simulink model "SZAU"  (R2017b)
settings: Solver=VariableStepAuto  StartTime=0.0  StopTime=1000  RelTol=1e-3
values from neighbouring files (symbols this model uses):
  A1 = 505    [SZAU_lin.mat]
  a1 = 22    [SZAU_lin.mat]
  a2 = 16    [SZAU_lin.mat]
  C2 = 0.65    [SZAU_lin.mat]
  Fd = 13    [SZAU_lin.mat]
  h10 = 17.87    [SZAU_lin.mat]
  h20 = 33.7852    [SZAU_lin.mat]
  tau = 80    [SZAU_lin.mat]
libraries: mpclib x1
settings Model: Creator=Jarzyn  LastModifiedBy=Jarzyn

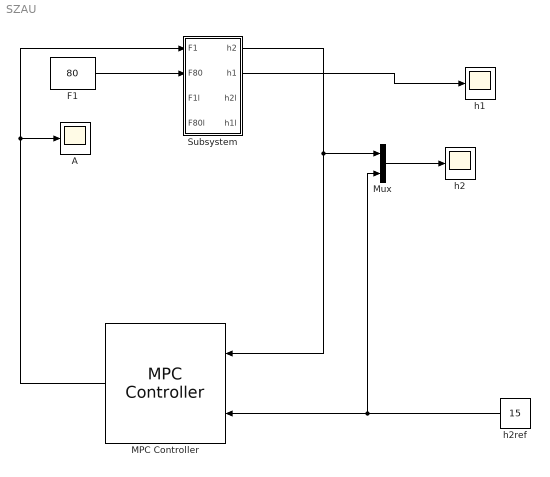
== system SZAU ==
  A : Scope
  F1 : Constant  Value=80  SampleTime=0
  MPC Controller : mpclib/MPC Controller  SCDEnableBlockLinearizationSpecification=on  mpcobj=mpc1  is_multiple=0  enable_value=0  return_u0=off  ref_from_ws=off  ref_signal_name=[]  ref_preview=off  md_from_ws=off  md_signal_name=[]  md_preview=off  from_project=off  project_file=MPCtask.mat  md_inport=off  mv_inport=off  cost_outport=off  return_sequence=off  return_qpstatus=off  return_state=off  state_inport=off  lims_inport=off  cc_inport=off  ywt_inport=off  is_designfromscratch=0  uwt_inport=off  duwt_inport=off  rhoeps_inport=off  uref_inport=off  n_ts=1  n_p=120  n_mv=1  n_md=0  n_ud=0  n_mo=1  n_uo=0  BlockDataType=double  SampleTimeInherited=off  switch_inport=off
  Mux : Mux  Inputs=2
  Subsystem : Subsystem
  h1 : Scope
  h2 : Scope
  h2ref : Constant  Value=15
  wires:
  Subsystem/1(h2) -> MPC Controller/1, Mux/1
  h2ref/1 -> Mux/2, MPC Controller/2
  Mux/1 -> h2/1
  Subsystem/2(h1) -> h1/1
  MPC Controller/1 -> A/1, Subsystem/1(F1)
  F1/1 -> Subsystem/2(F80)

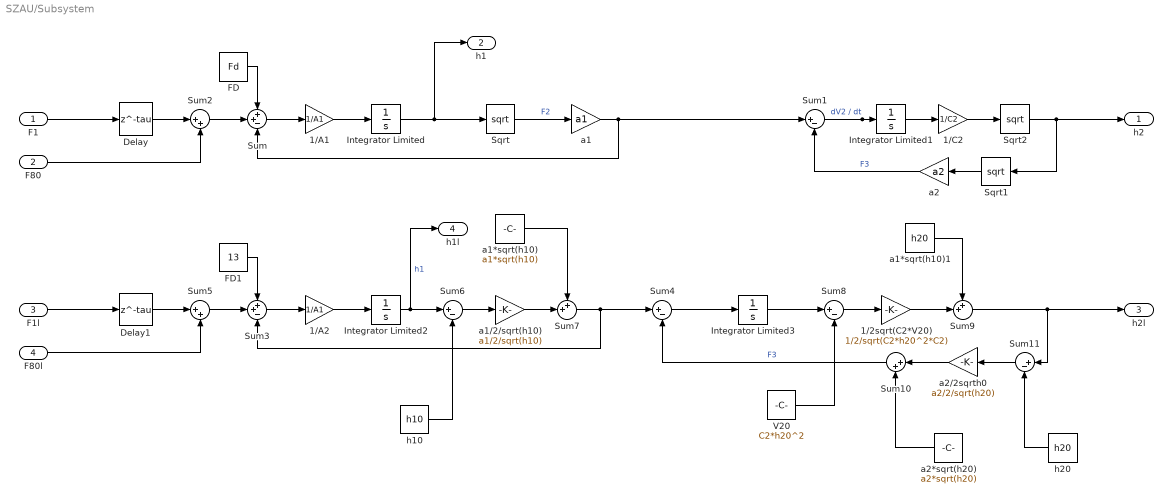
== system SZAU/Subsystem ==
  F1 : Inport
  F80 : Inport  Port=2
  F1l : Inport  Port=3
  F80l : Inport  Port=4
  1/2sqrt(C2*V20) : Gain  Gain=1/2/sqrt(C2*h20^2*C2)
  1/A1 : Gain  Gain=1/A1
  1/A2 : Gain  Gain=1/A1
  1/C2 : Gain  Gain=1/C2
  Delay : Delay  DelayLength=tau  InitialCondition=0
  Delay1 : Delay  DelayLength=tau  InitialCondition=0
  FD : Constant  Value=Fd
  FD1 : Constant  Value=13
  Integrator Limited : Integrator  InitialCondition=17.87  LimitOutput=on  LowerSaturationLimit=0
  Integrator Limited1 : Integrator  InitialCondition=0.65*33.7852^2  LimitOutput=on  LowerSaturationLimit=0
  Integrator Limited2 : Integrator  InitialCondition=h10  LimitOutput=on  LowerSaturationLimit=0
  Integrator Limited3 : Integrator  InitialCondition=C2*h20^2  LimitOutput=on  LowerSaturationLimit=0
  Sqrt : Sqrt  SaturateOnIntegerOverflow=on
  Sqrt1 : Sqrt  SaturateOnIntegerOverflow=on
  Sqrt2 : Sqrt  SaturateOnIntegerOverflow=on
  Sum : Sum  Inputs=++-
  Sum{1,4,6,8,11} (5 alike) : Sum  Inputs=|+-
  Sum10 : Sum  Inputs=|++
  Sum2 : Sum  Inputs=|++
  Sum3 : Sum  Inputs=++-
  Sum5 : Sum  Inputs=|++
  Sum7 : Sum  Inputs=++|
  Sum9 : Sum  Inputs=++|
  V20 : Constant  Value=C2*h20^2
  a1 : Gain  Gain=a1
  a1*sqrt(h10) : Constant  Value=a1*sqrt(h10)
  a1*sqrt(h10)1 : Constant  Value=h20
  a1/2/sqrt(h10) : Gain  Gain=a1/2/sqrt(h10)
  a2 : Gain  Gain=a2
  a2*sqrt(h20) : Constant  Value=a2*sqrt(h20)
  a2/2sqrth0 : Gain  Gain=a2/2/sqrt(h20)
  h10 : Constant  Value=h10
  h20 : Constant  Value=h20
  h2 : Outport
  h1 : Outport  Port=2
  h2l : Outport  Port=3
  h1l : Outport  Port=4
  wires:
  F1/1 -> Delay/1
  Sqrt1/1 -> a2/1
  FD/1 -> Sum/1
  Sum/1 -> 1/A1/1
  1/A1/1 -> Integrator Limited/1
  Sum1/1 -> Integrator Limited1/1  "dV2 / dt"
  Sqrt2/1 -> Sqrt1/1, h2/1
  a2/1 -> Sum1/2  "F3"
  Integrator Limited/1 -> h1/1, Sqrt/1
  Sqrt/1 -> a1/1  "F2"
  a1/1 -> Sum/3, Sum1/1
  Integrator Limited1/1 -> 1/C2/1
  F80/1 -> Sum2/2
  Delay/1 -> Sum2/1
  Sum2/1 -> Sum/2
  1/C2/1 -> Sqrt2/1
  Integrator Limited2/1 -> Sum6/1, h1l/1  "h1"
  Sum4/1 -> Integrator Limited3/1
  F80l/1 -> Sum5/2
  Sum5/1 -> Sum3/2
  Sum9/1 -> Sum11/1, h2l/1
  Delay1/1 -> Sum5/1
  Sum3/1 -> 1/A2/1
  F1l/1 -> Delay1/1
  FD1/1 -> Sum3/1
  1/A2/1 -> Integrator Limited2/1
  Integrator Limited3/1 -> Sum8/1
  h10/1 -> Sum6/2
  Sum6/1 -> a1/2/sqrt(h10)/1
  a1*sqrt(h10)/1 -> Sum7/1
  a1/2/sqrt(h10)/1 -> Sum7/2
  Sum7/1 -> Sum4/1, Sum3/3
  V20/1 -> Sum8/2
  a1*sqrt(h10)1/1 -> Sum9/1
  Sum8/1 -> 1/2sqrt(C2*V20)/1
  1/2sqrt(C2*V20)/1 -> Sum9/2
  h20/1 -> Sum11/2
  Sum11/1 -> a2/2sqrth0/1
  a2/2sqrth0/1 -> Sum10/1
  Sum10/1 -> Sum4/2  "F3"
  a2*sqrt(h20)/1 -> Sum10/2
